simulink model "TwoES10"  (R2017a)
settings: Solver=VariableStepAuto  StartTime=0.0  StopTime=10.0  MaxStep=1e-4  RelTol=1e-3
libraries: eltreclib x6, powerlib x3
settings Model: Creator=mayartmal  LastModifiedBy=mayartmal

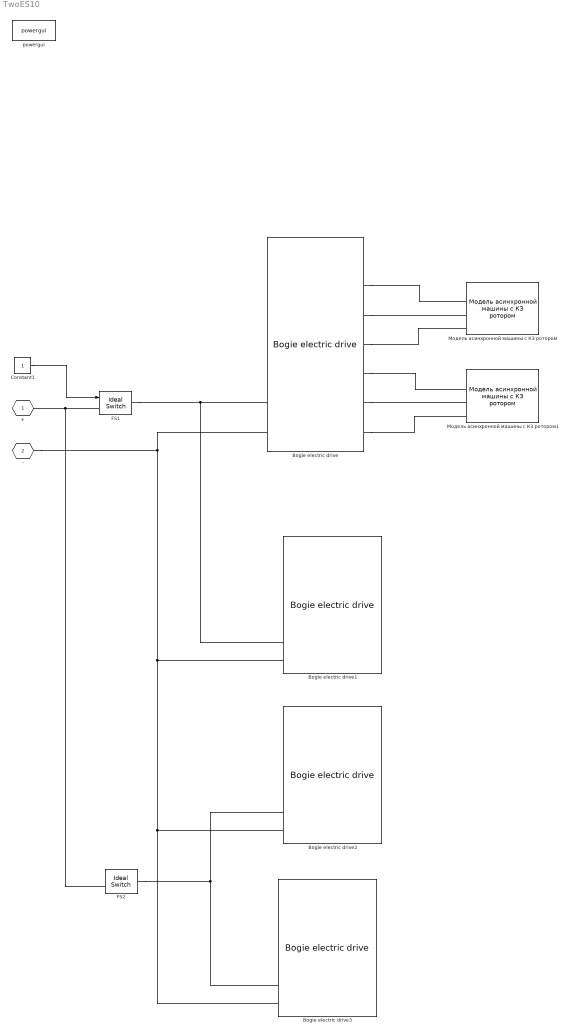
== system TwoES10 ==
  Bogie electric drive{,1..3} (4 alike) : eltreclib/Преобразователи 2ЭС10/Bogie electric drive
      settings: SourceProductName=Electric Traction
  Constant1 : Constant
  FS1 : powerlib/Power Electronics/Ideal Switch  Ron=0.001  Lon=0  IC=0  Rs=1e6  Cs=inf  Measurements=off
  FS2 : powerlib/Power Electronics/Ideal Switch  Ron=0.001  Lon=0  IC=0  Rs=1e6  Cs=inf  Measurements=off
  powergui : powerlib/powergui  Priority=1  SimulationMode=Continuous  SampleTime=50e-6  frequency=60  Iterations=50  frequencyindice=60  Pbase=100e6  ErrMax=1e-4  UnitsV=kV  UnitsW=MW  buscounter=0  FunctionMessages=off  echomessages=off  EnableUseOfTLC=off  CurrentSourceSwitches=off  DisableSnubberDevices=off  DisableRonSwitches=off  DisableVfSwitches=off  DisplayEquations=off  SolverType=Tustin/Backward Euler (TBE)  Interpol=off  ExternalGateDelay=off  methode=off  Ts=100  x0status=blocks  SPID=on  SwTol=0  HookPort=off  RestoreLinks=warning  ResistiveCurrentMeasurement=off  Frange=[0:2:500]  Ylog=off  Xlog=on  ShowGrid=off  save=off  variable=ZData  structure=0  ZoomFFT=off  StartTime=0.0  cycles=1  DisplayStyle=1  fundamental=60  FreqAxis=off  MaxFrequency=1000  frequencyindicesteady=1  RmsSteady=1  display=off
  Модель асинхронной машины с КЗ ротором : eltreclib/Модель асинхронной машины с КЗ ротором  f_nominal=50  Rs=0.0472  ls=0.0003883  Rr=0.0392  lr=0.0005399  Lm=0.011  Zp=2
      settings: SourceProductName=Electric Traction
  Модель асинхронной машины с КЗ ротором1 : eltreclib/Модель асинхронной машины с КЗ ротором  f_nominal=50  Rs=0.0472  ls=0.0003883  Rr=0.0392  lr=0.0005399  Lm=0.011  Zp=2
      settings: SourceProductName=Electric Traction
  + : PMIOPort  Tag=PMCPort  Port=1  Side=Left
  - : PMIOPort  Tag=PMCPort  Port=2  Side=Left
  wires:
  Constant1/1 -> FS1/1
  connections:
  FS1/LConn1 -- FS2/LConn1 -- +/RConn1
  -/RConn1 -- Bogie electric drive1/LConn2 -- Bogie electric drive3/LConn2 -- Bogie electric drive2/LConn2 -- Bogie electric drive/LConn2
  FS1/RConn1 -- Bogie electric drive1/LConn1 -- Bogie electric drive/LConn1
  FS2/RConn1 -- Bogie electric drive2/LConn1 -- Bogie electric drive3/LConn1
  Bogie electric drive/RConn1 -- Модель асинхронной машины с КЗ ротором/LConn1
  Bogie electric drive/RConn2 -- Модель асинхронной машины с КЗ ротором/LConn2
  Bogie electric drive/RConn3 -- Модель асинхронной машины с КЗ ротором/LConn3
  Bogie electric drive/RConn4 -- Модель асинхронной машины с КЗ ротором1/LConn1
  Bogie electric drive/RConn5 -- Модель асинхронной машины с КЗ ротором1/LConn2
  Bogie electric drive/RConn6 -- Модель асинхронной машины с КЗ ротором1/LConn3
